simulink library "PhaseCheck"  (R2018b)
settings: Solver=ode45  StartTime=0.0  StopTime=10.0  RelTol=1e-3  EnableMultiTasking=on
libraries: carnot x1
settings Model: Creator=lena.frank  LastModifiedBy=drhf
settings DataIOCC: LimitDataPoints=on  SaveFormat=Array  SignalLoggingSaveFormat=ModelDataLogs
settings OptimizationCC: ExpressionDepthLimit=2147483647  LifeSpan=inf
settings DebuggingCC: UnderspecifiedInitializationDetection=Classic  MergeDetectMultiDrivingBlocksExec=none  SolverPrmCheckMsg=warning  FcnCallInpInsideContextMsg=warning  StateNameClashWarn=warning  SFUnexpectedBacktrackingDiag=warning  SFNoUnconditionalDefaultTransitionDiag=warning  SFExecutionAtInitializationDiag=none
settings HardwareCC: ProdBitPerPointer=32  ProdBitPerSizeT=32  ProdBitPerPtrDiffT=32  ProdLargestAtomicFloat=None  ProdIntDivRoundTo=Undefined  ProdEndianess=Unspecified  ProdWordSize=32  ProdHWDeviceType=32-bit Generic
settings ModelReferenceCC: PropagateSignalLabelsOutOfModel=off
settings SFSimCC: SimUseLocalCustomCode=off
settings RTWCC: RTWUseLocalCustomCode=off
settings CodeAppCC: StateflowObjectComments=on
settings GRTTargetCC: TargetLangStandard=C89/C90 (ANSI)  GeneratePreprocessorConditionals=Disable all  CombineOutputUpdateFcns=off  GRTInterface=on
settings ConfigComp: CovMetricSettings=dw  CovHtmlReporting=on  CovSaveCumulativeToWorkspaceVar=on  CovSaveSingleToWorkspaceVar=on  CovExternalEMLEnable=off

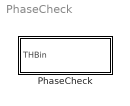
== system PhaseCheck ==
  PhaseCheck : Subsystem  mask(phasecheck){}
      mask help: Checks whether fluid is still in the correct phase, for example if water is not steam or ice. Simulation is stopped for inconstistent phase.
      mask Help: web(fullfile(path_carnot('help'),'PhaseCheck.html'),'-helpbrowser')

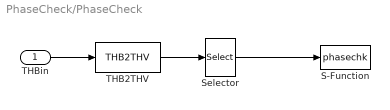
== system PhaseCheck/PhaseCheck ==
  THBin : Inport
  S-Function : S-Function  FunctionName=phasechk  SFunctionDeploymentMode=off  EnableBusSupport=off
  Selector : Selector  InputPortWidth=20  IndexOptions=Index vector (dialog)  Indices=[2:6]  OutputSizes=1
  THB2THV : carnot/Toolbox/THB2THV
      settings: SourceProductName=Carnot
  wires:
  THB2THV/1 -> Selector/1
  THBin/1 -> THB2THV/1
  Selector/1 -> S-Function/1
